simulink model "process"  (R2018b)
settings: Solver=ode45  StartTime=0.0  StopTime=Ts  RelTol=1e-8  EnableMultiTasking=on
values from neighbouring files (symbols this model uses):
  A = [(sin(th1)-sin(th1+2*th2))/(-3+cos(2*th2))  , (-sin(th1)+3*sin(th1+th2)-sin(th1-th2)+sin(th1+2*th2))/(-3+cos(2*th2)) ... (first row only)    [ajuda.m]    (also in controledesacoplante.m; gazebo_parameters.m = Amd; geracao.m = 0; gpc.m = [1.0013 0 0.0050)
  B = Bmd    [gazebo_parameters.m]    (also in geracao.m = 1; gpc.m = [-0.001; kalman_filter.m; questao1.m = double(subs(u, [x1 x2],[0 0])))
  x0 = [pi/180*45 0 0]    [questao1.m]
undefined symbols (not defined in the file or in its folder): U, Um1
settings Model: Creator=julioelias  LastModifiedBy=root
settings DataIOCC: LimitDataPoints=on  SaveFormat=Array  SignalLoggingSaveFormat=ModelDataLogs  TimeSaveName=tempo
settings OptimizationCC: LifeSpan=inf
settings DebuggingCC: SaveWithParameterizedLinksMsg=none  UnderspecifiedInitializationDetection=Classic  MergeDetectMultiDrivingBlocksExec=none  FcnCallInpInsideContextMsg=warning  StateNameClashWarn=warning  SFUnexpectedBacktrackingDiag=warning  SFNoUnconditionalDefaultTransitionDiag=warning  SFExecutionAtInitializationDiag=none
settings HardwareCC: ProdBitPerPointer=32  ProdBitPerSizeT=32  ProdBitPerPtrDiffT=32  ProdLargestAtomicFloat=None  ProdIntDivRoundTo=Undefined  ProdEndianess=Unspecified  ProdWordSize=32  ProdHWDeviceType=32-bit Generic
settings ModelReferenceCC: PropagateSignalLabelsOutOfModel=off
settings SFSimCC: SimUseLocalCustomCode=off
settings RTWCC: RTWUseLocalCustomCode=off
settings CodeAppCC: StateflowObjectComments=on
settings GRTTargetCC: TargetLangStandard=C89/C90 (ANSI)  CodeReplacementLibrary=NOT IN USE  GeneratePreprocessorConditionals=Disable all  CombineOutputUpdateFcns=off  GRTInterface=on
settings ConfigComp: CovMetricSettings=dw  CovHtmlReporting=on  CovSaveCumulativeToWorkspaceVar=on  CovSaveSingleToWorkspaceVar=on  CovExternalEMLEnable=off

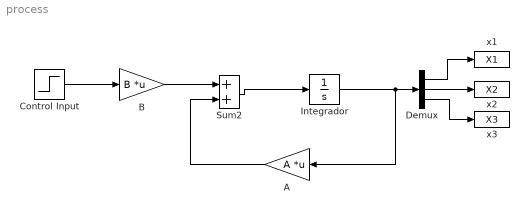
== system process ==
  "A " : Gain  Gain=A  Multiplication=Matrix(K*u)  SaturateOnIntegerOverflow=on  OutDataTypeStr=Inherit: Same as input  ParamDataTypeStr=Inherit: Same as input
  B : Gain  Gain=B  Multiplication=Matrix(K*u)  SaturateOnIntegerOverflow=on  OutDataTypeStr=Inherit: Same as input  ParamDataTypeStr=Inherit: Same as input
  Control Input : Step  Time=0  Before=Um1  After=U  SampleTime=0
  Demux : Demux  Outputs=3
  Integrador : Integrator  InitialCondition=x0
  Sum2 : Sum  SaturateOnIntegerOverflow=on  InputSameDT=on  OutDataTypeStr=Inherit: Same as first input
  x1 : ToWorkspace  VariableName=X1  SampleTime=-1
  x2 : ToWorkspace  VariableName=X2  SampleTime=-1
  x3 : ToWorkspace  VariableName=X3  SampleTime=-1
  wires:
  Sum2/1 -> Integrador/1
  Integrador/1 -> Demux/1, "A "/1
  Control Input/1 -> B/1
  B/1 -> Sum2/1
  "A "/1 -> Sum2/2
  Demux/3 -> x3/1
  Demux/2 -> x2/1
  Demux/1 -> x1/1
